simulink subsystem "SystemControl"  (R2019b)
settings: Solver=VariableStepAuto  StartTime=0.0  StopTime=10.0  RelTol=1e-3
undefined symbols (not defined in the file): etcModes, motorControlModes, motorPosGainI, motorPosGainP, motorVelGainFeedback, motorVelGainI, motorVelGainP, throttlePosInputModes
libraries: simulink x10, FunctionCallDivider x2
settings Model: Creator=Nick  LastModifiedBy=Nick

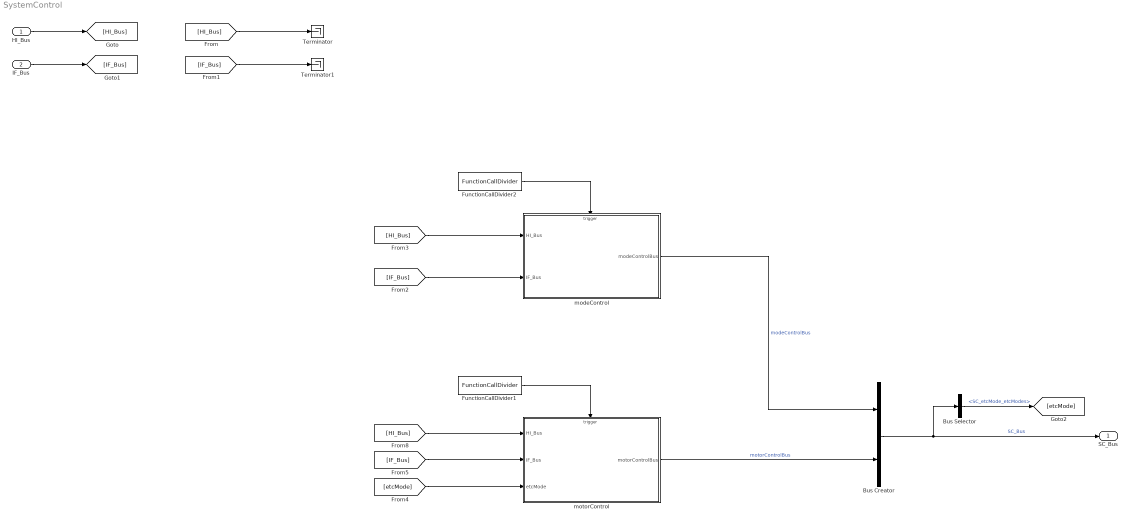
== system SystemControl ==
  HI_Bus : Inport
  IF_Bus : Inport  Port=2
  Bus Creator : BusCreator  Inputs=2
  Bus Selector : BusSelector  OutputSignals=modeControlBus.SC_etcMode_etcModes
  FunctionCallDivider1 : FunctionCallDivider/Algroithms/FunctionCallDivider  counts=1
  FunctionCallDivider2 : FunctionCallDivider/Algroithms/FunctionCallDivider  counts=10
  Terminator : Terminator
  Terminator1 : Terminator
  modeControl : Subsystem  TreatAsAtomicUnit=on
  motorControl : Subsystem  TreatAsAtomicUnit=on
  SC_Bus : Outport
  wires:
  IF_Bus/1 -> [IF_Bus]
  Bus Creator/1 -> SC_Bus/1, Bus Selector/1  "SC_Bus"
  [HI_Bus] -> Terminator/1
  [IF_Bus] -> Terminator1/1
  HI_Bus/1 -> [HI_Bus]
  [HI_Bus] -> motorControl/1(HI_Bus)
  FunctionCallDivider1/1 -> motorControl/Trigger
  [IF_Bus] -> motorControl/2(IF_Bus)
  motorControl/1(motorControlBus) -> Bus Creator/2  "motorControlBus"
  [IF_Bus] -> modeControl/2(IF_Bus)
  FunctionCallDivider2/1 -> modeControl/Trigger
  [HI_Bus] -> modeControl/1(HI_Bus)
  modeControl/1(modeControlBus) -> Bus Creator/1  "modeControlBus"
  Bus Selector/1 -> [etcMode]  "<SC_etcMode_etcModes>"
  [etcMode] -> motorControl/3(etcMode)

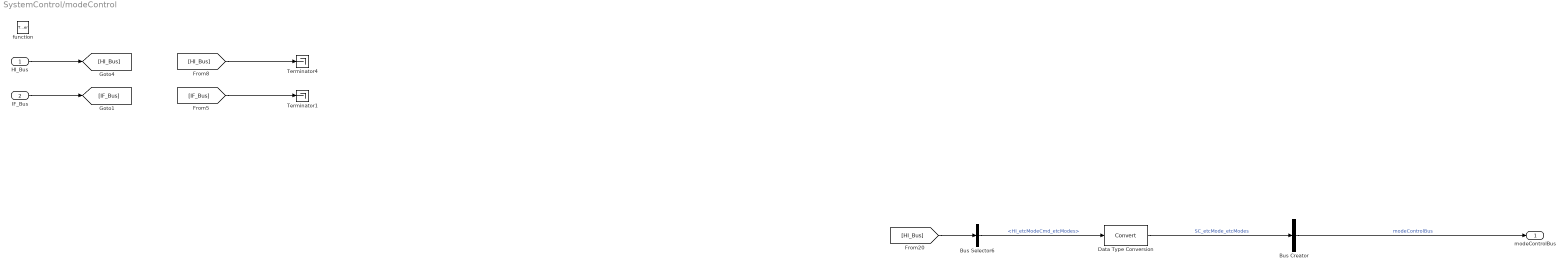
== system SystemControl/modeControl ==
  HI_Bus : Inport
  IF_Bus : Inport  Port=2
  function : TriggerPort  TriggerType=function-call  VariantControl=Variant
  Bus Creator : BusCreator  Inputs=1
  Bus Selector6 : BusSelector  OutputSignals=VectorBoxBus.HI_etcModeCmd_etcModes
  Data Type Conversion : DataTypeConversion
  Terminator1 : Terminator
  Terminator4 : Terminator
  modeControlBus : Outport
  wires:
  Data Type Conversion/1 -> Bus Creator/1  "SC_etcMode_etcModes"
  Bus Selector6/1 -> Data Type Conversion/1  "<HI_etcModeCmd_etcModes>"
  [HI_Bus] -> Bus Selector6/1
  Bus Creator/1 -> modeControlBus/1  "modeControlBus"
  [IF_Bus] -> Terminator1/1
  HI_Bus/1 -> [HI_Bus]
  [HI_Bus] -> Terminator4/1
  IF_Bus/1 -> [IF_Bus]

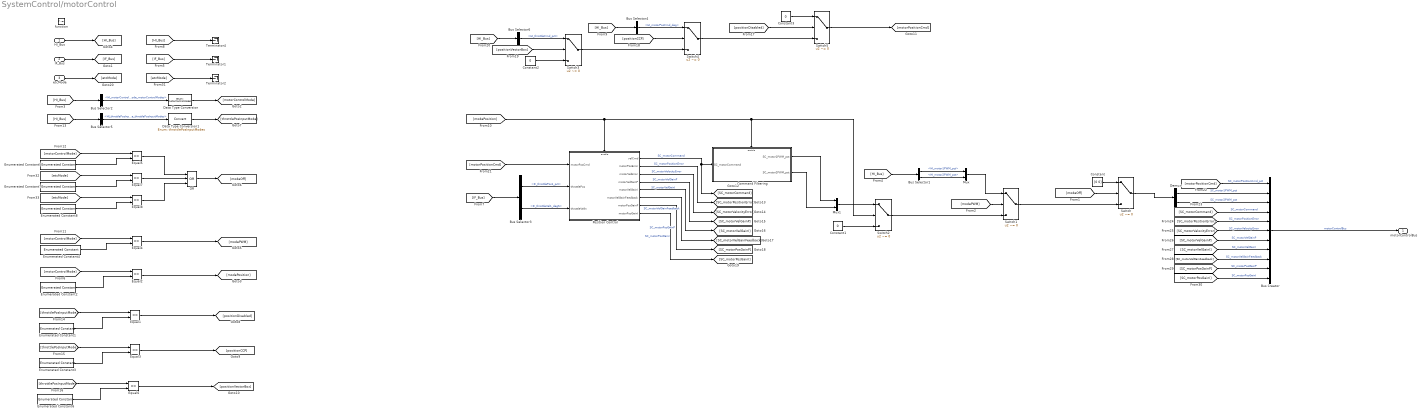
== system SystemControl/motorControl ==
  HI_Bus : Inport
  IF_Bus : Inport  Port=2
  etcMode : Inport  Port=3
  function : TriggerPort  TriggerType=function-call  VariantControl=Variant
  Bus Creator : BusCreator  Inputs=11
  Bus Selector1 : BusSelector  OutputSignals=VectorBoxBus.HI_motor1PWM_pct,VectorBoxBus.HI_motor2PWM_pct
  Bus Selector2 : BusSelector  OutputSignals=VectorBoxBus.HI_motorControlMode_motorControlModes
  Bus Selector3 : BusSelector  OutputSignals=AnalogInputFiltering_Bus.ExternalADCBus.IF_throttlePos1_pct,AnalogInputFiltering_Bus.ExternalADCBus.IF_throttleVel1_degS
  Bus Selector4 : BusSelector  OutputSignals=VectorBoxBus.HI_motorPosCmd_deg
  Bus Selector5 : BusSelector  OutputSignals=VectorBoxBus.HI_throttlePosInputMode_throttlePosInputModes
  Bus Selector6 : BusSelector  OutputSignals=VectorBoxBus.HI_throttleCmd_pct
  Command Filtering : Subsystem
  Constant : Constant  Value=[0 0]
  Constant1 : Constant  Value=0
  Constant2 : Constant  Value=0
  Constant3 : Constant  Value=0
  Data Type Conversion : DataTypeConversion  OutDataTypeStr=Enum: motorControlModes
  Data Type Conversion1 : DataTypeConversion  OutDataTypeStr=Enum: throttlePosInputModes
  Demux : Demux  Outputs=2
  Enumerated Constant1 : simulink/Sources/Enumerated Constant  OutDataTypeStr=Enum: throttlePosInputModes  Value=throttlePosInputModes.Disabled  SampleTime=inf
      settings: SourceProductName=Simulink
  Enumerated Constant2 : simulink/Sources/Enumerated Constant  OutDataTypeStr=Enum: motorControlModes  Value=motorControlModes.Position  SampleTime=inf
      settings: SourceProductName=Simulink
  Enumerated Constant3 : simulink/Sources/Enumerated Constant  OutDataTypeStr=Enum: throttlePosInputModes  Value=throttlePosInputModes.CCP  SampleTime=inf
      settings: SourceProductName=Simulink
  Enumerated Constant4 : simulink/Sources/Enumerated Constant  OutDataTypeStr=Enum: motorControlModes  Value=motorControlModes.PWM  SampleTime=inf
      settings: SourceProductName=Simulink
  Enumerated Constant5 : simulink/Sources/Enumerated Constant  OutDataTypeStr=Enum: motorControlModes  Value=motorControlModes.Off  SampleTime=inf
      settings: SourceProductName=Simulink
  Enumerated Constant6 : simulink/Sources/Enumerated Constant  OutDataTypeStr=Enum: throttlePosInputModes  Value=throttlePosInputModes.VectorBox  SampleTime=inf
      settings: SourceProductName=Simulink
  Enumerated Constant7 : simulink/Sources/Enumerated Constant  OutDataTypeStr=Enum: etcModes  Value=etcModes.ESTOP  SampleTime=inf
      settings: SourceProductName=Simulink
  Enumerated Constant8 : simulink/Sources/Enumerated Constant  OutDataTypeStr=Enum: etcModes  Value=etcModes.Standby  SampleTime=inf
      settings: SourceProductName=Simulink
  Equal{1..8} (8 alike) : RelationalOperator  Operator===  OutDataTypeStr=boolean  RndMeth=Simplest
  Mux : Mux  Inputs=2
  Mux1 : Mux  Inputs=2
  OR : Logic  Operator=OR  Inputs=3  IconShape=distinctive  AllPortsSameDT=off  OutDataTypeStr=boolean
  Position Control : Subsystem  TreatAsAtomicUnit=on
  Switch{,1..5} (6 alike) : Switch  Criteria=u2 ~= 0
  Terminator1 : Terminator
  Terminator2 : Terminator
  Terminator4 : Terminator
  motorControlBus : Outport
  wires:
  Equal8/1 -> OR/3
  Equal7/1 -> OR/2
  [etcMode] -> Equal8/1
  Enumerated Constant8/1 -> Equal8/2
  OR/1 -> [modeOff]
  [etcMode] -> Equal7/1
  Enumerated Constant7/1 -> Equal7/2
  [etcMode] -> Terminator2/1
  etcMode/1 -> [etcMode]
  [SC_motorVelGainP] -> Bus Creator/7  "SC_motorVelGainP"
  [SC_motorVelGainI] -> Bus Creator/8  "SC_motorVelGainI"
  [SC_motorVelGainFeedback] -> Bus Creator/9  "SC_motorVelGainFeedback"
  [SC_motorPosGainP] -> Bus Creator/10  "SC_motorPosGainP"
  [SC_motorPosGainI] -> Bus Creator/11  "SC_motorPosGainI"
  Position Control/8(motorPosGainI) -> [SC_motorPosGainI]  "SC_motorPosGainI"
  Position Control/7(motorPosGainP) -> [SC_motorPosGainP]  "SC_motorPosGainP"
  Position Control/6(motorVelGainFeedback) -> [SC_motorVelGainFeedback]  "SC_motorVelGainFeedback"
  Position Control/5(motorVelGainI) -> [SC_motorVelGainI]  "SC_motorVelGainI"
  Position Control/4(motorVelGainP) -> [SC_motorVelGainP]  "SC_motorVelGainP"
  [SC_motorCommand] -> Bus Creator/4  "SC_motorCommand"
  [SC_motorPositionError] -> Bus Creator/5  "SC_motorPositionError"
  [SC_motorVelocityError] -> Bus Creator/6  "SC_motorVelocityError"
  Position Control/3(motorVelError) -> [SC_motorVelocityError]  "SC_motorVelocityError"
  Position Control/2(motorPosError) -> [SC_motorPositionError]  "SC_motorPositionError"
  [motorPositionCmd] -> Bus Creator/1  "SC_motorPositionCmd_pct"
  [motorPositionCmd] -> Position Control/1(motorPosCmd)
  Switch5/1 -> [motorPositionCmd]
  [HI_Bus] -> Bus Selector6/1
  Bus Selector6/1 -> Switch3/1  "<HI_throttleCmd_pct>"
  Bus Selector4/1 -> Switch4/1  "<HI_motorPosCmd_deg>"
  [HI_Bus] -> Bus Selector4/1
  [positionVectorBox] -> Switch3/2
  [positionCCP] -> Switch4/2
  [positionDisabled] -> Switch5/2
  Constant3/1 -> Switch5/1
  Constant2/1 -> Switch3/3
  [throttlePosInputMode] -> Equal6/1
  Enumerated Constant6/1 -> Equal6/2
  Equal6/1 -> [positionVectorBox]
  [throttlePosInputMode] -> Equal3/1
  Enumerated Constant3/1 -> Equal3/2
  Equal3/1 -> [positionCCP]
  [throttlePosInputMode] -> Equal1/1
  Enumerated Constant1/1 -> Equal1/2
  Equal1/1 -> [positionDisabled]
  Data Type Conversion1/1 -> [throttlePosInputMode]
  [HI_Bus] -> Bus Selector5/1
  Bus Selector5/1 -> Data Type Conversion1/1  "<HI_throttlePosInputMode_throttlePosInputModes>"
  Switch4/1 -> Switch5/3
  Switch3/1 -> Switch4/3
  Equal5/1 -> OR/1
  [motorControlMode] -> Equal5/1
  Enumerated Constant5/1 -> Equal5/2
  Equal4/1 -> [modePWM]
  Enumerated Constant4/1 -> Equal4/2
  [motorControlMode] -> Equal4/1
  Equal2/1 -> [modePosition]
  [motorControlMode] -> Equal2/1
  Enumerated Constant2/1 -> Equal2/2
  Command Filtering/2(SC_motor2PWM_pct) -> Mux1/2
  Command Filtering/1(SC_motor1PWM_pct) -> Mux1/1
  Bus Selector3/1 -> Position Control/2(throttlePos)  "<IF_throttlePos1_pct>"
  Bus Selector3/2 -> Position Control/3(throttleVelIn)  "<IF_throttleVel1_degS>"
  Position Control/1(velCmd) -> Command Filtering/1(SC_motorCommand), [SC_motorCommand]  "SC_motorCommand"
  [modePosition] -> Position Control/Enable, Switch2/2, Command Filtering/Enable
  [IF_Bus] -> Bus Selector3/1
  Constant1/1 -> Switch2/3
  Switch2/1 -> Switch1/3
  Mux1/1 -> Switch2/1
  Bus Selector1/2 -> Mux/2  "<HI_motor2PWM_pct>"
  Bus Selector1/1 -> Mux/1  "<HI_motor1PWM_pct>"
  [HI_Bus] -> Bus Selector1/1
  Mux/1 -> Switch1/1
  Data Type Conversion/1 -> [motorControlMode]
  [HI_Bus] -> Bus Selector2/1
  Bus Selector2/1 -> Data Type Conversion/1  "<HI_motorControlMode_motorControlModes>"
  [modePWM] -> Switch1/2
  Switch1/1 -> Switch/3
  Constant/1 -> Switch/1
  [modeOff] -> Switch/2
  Demux/2 -> Bus Creator/3  "SC_motor2PWM_pct"
  Demux/1 -> Bus Creator/2  "SC_motor1PWM_pct"
  Switch/1 -> Demux/1
  Bus Creator/1 -> motorControlBus/1  "motorControlBus"
  [IF_Bus] -> Terminator1/1
  HI_Bus/1 -> [HI_Bus]
  [HI_Bus] -> Terminator4/1
  IF_Bus/1 -> [IF_Bus]

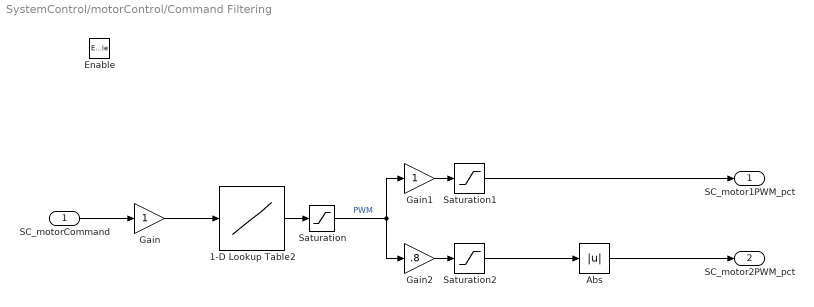
== system SystemControl/motorControl/Command Filtering ==
  SC_motorCommand : Inport
  Enable : EnablePort  StatesWhenEnabling=reset
  1-D Lookup Table2 : Lookup_n-D  NumberOfTableDimensions=1  BreakpointsForDimension1=[-100 -5 -.1 0 .1 5 100]  Table=[-100 -5 -1 0 1 20 100]  InternalRulePriority=Speed  RndMeth=Simplest  InputSameDT=on
  Abs : Abs
  Gain : Gain
  Gain1 : Gain
  Gain2 : Gain  Gain=.8
  Saturation : Saturate  UpperLimit=100  LowerLimit=-100
  Saturation1 : Saturate  UpperLimit=100  LowerLimit=0
  Saturation2 : Saturate  UpperLimit=0  LowerLimit=-100
  SC_motor1PWM_pct : Outport
  SC_motor2PWM_pct : Outport  Port=2
  wires:
  Abs/1 -> SC_motor2PWM_pct/1
  1-D Lookup Table2/1 -> Saturation/1
  Gain/1 -> 1-D Lookup Table2/1
  Saturation2/1 -> Abs/1
  Gain1/1 -> Saturation1/1
  Gain2/1 -> Saturation2/1
  SC_motorCommand/1 -> Gain/1
  Saturation/1 -> Gain1/1, Gain2/1  "PWM"
  Saturation1/1 -> SC_motor1PWM_pct/1

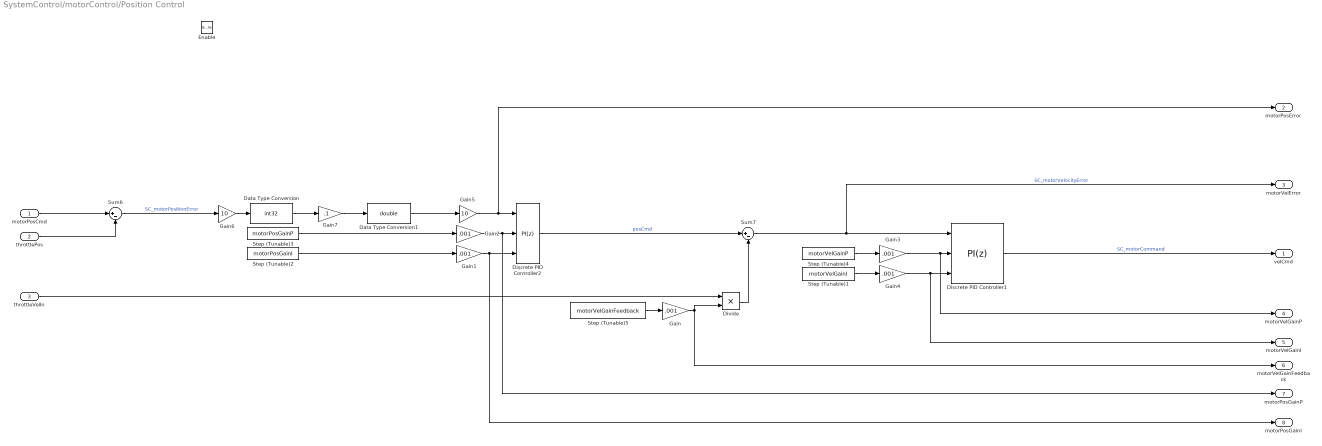
== system SystemControl/motorControl/Position Control ==
  motorPosCmd : Inport
  throttlePos : Inport  Port=2
  throttleVelIn : Inport  Port=3
  Enable : EnablePort  StatesWhenEnabling=reset
  Data Type Conversion : DataTypeConversion  OutDataTypeStr=int32
  Data Type Conversion1 : DataTypeConversion  OutDataTypeStr=double
  Discrete PID Controller1 : simulink/Continuous/PID Controller  Controller=PI  Form=Ideal  TimeDomain=Discrete-time  SampleTime=-1  IntegratorMethod=Forward Euler  FilterMethod=Forward Euler  ControllerParametersSource=external  P=0  I=0  D=0  UseFilter=off  N=100  TunerSelectOption=Transfer Function Based (PID Tuner App)  InitialConditionSource=internal  InitialConditionForIntegrator=0  InitialConditionForFilter=0  DifferentiatorICPrevScaledInput=0  ExternalReset=none  TrackingMode=off  Kt=1  LimitOutput=on  UpperSaturationLimit=100  LowerSaturationLimit=-100  LinearizeAsGain=off  AntiWindupMode=none  Kb=1  POutMin=[]  POutMax=[]  IOutMin=[]  IOutMax=[]  DOutMin=[]  DOutMax=[]  NOutMin=[]  NOutMax=[]  SumOutMin=[]  SumOutMax=[]  SaturationOutMin=[]  SaturationOutMax=[]  PParamMin=[]  PParamMax=[]  IParamMin=[]  IParamMax=[]  DParamMin=[]  DParamMax=[]  NParamMin=[]  NParamMax=[]  KbParamMin=[]  KbParamMax=[]  KtParamMin=[]  KtParamMax=[]  KbOutMin=[]  KbOutMax=[]  KtOutMin=[]  KtOutMax=[]  IntegratorOutMin=[]  IntegratorOutMax=[]  FilterOutMin=[]  FilterOutMax=[]  SumI1OutMin=[]  SumI1OutMax=[]  SumI2OutMin=[]  SumI2OutMax=[]  SumI3OutMin=[]  SumI3OutMax=[]  SumI4OutMin=[]  SumI4OutMax=[]  SumDOutMin=[]  SumDOutMax=[]  DifferentiatorOutMin=[]  DifferentiatorOutMax=[]  FilterDiffOutCoefMin=[]  FilterDiffOutCoefMax=[]  ReciprocalOutMin=[]  ReciprocalOutMax=[]  SumDenOutMin=[]  SumDenOutMax=[]  SumNumOutMin=[]  SumNumOutMax=[]  DivideOutMin=[]  DivideOutMax=[]  IntegratorContinuousStateAttributes=''  IntegratorStateMustResolveToSignalObject=off  IntegratorRTWStateStorageClass=Auto  FilterContinuousStateAttributes=''  FilterStateMustResolveToSignalObject=off  FilterRTWStateStorageClass=Auto  ParallelPVariant=Passthrough  IdealPVariant=ExternalParameters  IVariant=ExternalParameters  DVariant=Disabled  IntegratorVariant=Discrete  SatVariant=Enabled  AWVariant=Passthrough  PCopyVariant=Disabled  TRVariant=Disabled  FdbkBlocksVariant=Forward  IdealPFdbkVariant=Disabled  SatFdbkVariant=Disabled  DerivativeFilterVariant=Disabled  NVariant=Disabled  NCopyVariant=Disabled_SignalSpec  FilterICVariant=Disabled  IntegratorICVariant=InternalICs  ExternalResetVariant=Disabled  TRSumVariant=Passthrough  SumFdbkVariant=Disabled  SumVariant=Sum_PI
  Discrete PID Controller2 : simulink/Continuous/PID Controller  Controller=PI  Form=Ideal  TimeDomain=Discrete-time  SampleTime=-1  IntegratorMethod=Forward Euler  FilterMethod=Forward Euler  ControllerParametersSource=external  P=0  I=0  D=0  UseFilter=off  N=100  TunerSelectOption=Transfer Function Based (PID Tuner App)  InitialConditionSource=internal  InitialConditionForIntegrator=0  InitialConditionForFilter=0  DifferentiatorICPrevScaledInput=0  ExternalReset=none  TrackingMode=off  Kt=1  LimitOutput=on  UpperSaturationLimit=500  LowerSaturationLimit=-500  LinearizeAsGain=off  AntiWindupMode=none  Kb=1  POutMin=[]  POutMax=[]  IOutMin=[]  IOutMax=[]  DOutMin=[]  DOutMax=[]  NOutMin=[]  NOutMax=[]  SumOutMin=[]  SumOutMax=[]  SaturationOutMin=[]  SaturationOutMax=[]  PParamMin=[]  PParamMax=[]  IParamMin=[]  IParamMax=[]  DParamMin=[]  DParamMax=[]  NParamMin=[]  NParamMax=[]  KbParamMin=[]  KbParamMax=[]  KtParamMin=[]  KtParamMax=[]  KbOutMin=[]  KbOutMax=[]  KtOutMin=[]  KtOutMax=[]  IntegratorOutMin=[]  IntegratorOutMax=[]  FilterOutMin=[]  FilterOutMax=[]  SumI1OutMin=[]  SumI1OutMax=[]  SumI2OutMin=[]  SumI2OutMax=[]  SumI3OutMin=[]  SumI3OutMax=[]  SumI4OutMin=[]  SumI4OutMax=[]  SumDOutMin=[]  SumDOutMax=[]  DifferentiatorOutMin=[]  DifferentiatorOutMax=[]  FilterDiffOutCoefMin=[]  FilterDiffOutCoefMax=[]  ReciprocalOutMin=[]  ReciprocalOutMax=[]  SumDenOutMin=[]  SumDenOutMax=[]  SumNumOutMin=[]  SumNumOutMax=[]  DivideOutMin=[]  DivideOutMax=[]  IntegratorContinuousStateAttributes=''  IntegratorStateMustResolveToSignalObject=off  IntegratorRTWStateStorageClass=Auto  FilterContinuousStateAttributes=''  FilterStateMustResolveToSignalObject=off  FilterRTWStateStorageClass=Auto  ParallelPVariant=Passthrough  IdealPVariant=ExternalParameters  IVariant=ExternalParameters  DVariant=Disabled  IntegratorVariant=Discrete  SatVariant=Enabled  AWVariant=Passthrough  PCopyVariant=Disabled  TRVariant=Disabled  FdbkBlocksVariant=Forward  IdealPFdbkVariant=Disabled  SatFdbkVariant=Disabled  DerivativeFilterVariant=Disabled  NVariant=Disabled  NCopyVariant=Disabled_SignalSpec  FilterICVariant=Disabled  IntegratorICVariant=InternalICs  ExternalResetVariant=Disabled  TRSumVariant=Passthrough  SumFdbkVariant=Disabled  SumVariant=Sum_PI
  Divide : Product  Inputs=**
  Gain{,1..4} (5 alike) : Gain  Gain=.001
  Gain5 : Gain  Gain=10
  Gain6 : Gain  Gain=10
  Gain7 : Gain  Gain=.1
  Step (Tunable)1 : Constant  Value=motorVelGainI  VectorParams1D=off  SampleTime=-1
  Step (Tunable)2 : Constant  Value=motorPosGainI  VectorParams1D=off  SampleTime=-1
  Step (Tunable)3 : Constant  Value=motorPosGainP  VectorParams1D=off  SampleTime=-1
  Step (Tunable)4 : Constant  Value=motorVelGainP  VectorParams1D=off  SampleTime=-1
  Step (Tunable)5 : Constant  Value=motorVelGainFeedback  VectorParams1D=off  SampleTime=-1
  Sum6 : Sum  Inputs=|+-
  Sum7 : Sum  Inputs=|+-
  velCmd : Outport
  motorPosError : Outport  Port=2
  motorVelError : Outport  Port=3
  motorVelGainP : Outport  Port=4
  motorVelGainI : Outport  Port=5
  motorVelGainFeedback : Outport  Port=6
  motorPosGainP : Outport  Port=7
  motorPosGainI : Outport  Port=8
  wires:
  Data Type Conversion1/1 -> Gain5/1
  Data Type Conversion/1 -> Gain7/1
  Gain7/1 -> Data Type Conversion1/1
  Gain6/1 -> Data Type Conversion/1
  Gain5/1 -> Discrete PID Controller2/1, motorPosError/1
  Gain4/1 -> Discrete PID Controller1/3, motorVelGainI/1
  Gain3/1 -> Discrete PID Controller1/2, motorVelGainP/1
  Gain2/1 -> Discrete PID Controller2/2, motorPosGainP/1
  Gain1/1 -> Discrete PID Controller2/3, motorPosGainI/1
  Gain/1 -> Divide/2, motorVelGainFeedback/1
  Step (Tunable)5/1 -> Gain/1
  Discrete PID Controller2/1 -> Sum7/1  "posCmd"
  Step (Tunable)4/1 -> Gain3/1
  Sum7/1 -> motorVelError/1, Discrete PID Controller1/1  "SC_motorVelocityError"
  Discrete PID Controller1/1 -> velCmd/1  "SC_motorCommand"
  throttleVelIn/1 -> Divide/1
  Step (Tunable)1/1 -> Gain4/1
  Divide/1 -> Sum7/2
  throttlePos/1 -> Sum6/2
  Step (Tunable)2/1 -> Gain1/1
  Step (Tunable)3/1 -> Gain2/1
  motorPosCmd/1 -> Sum6/1
  Sum6/1 -> Gain6/1  "SC_motorPositionError"
